simulink model "PlantaHinf"  (R2016a)
settings: Solver=ode45  StartTime=0.0  StopTime=inf  RelTol=1e-3
undefined symbols (not defined in the file or in its folder): K1
libraries: arduino_io_lib x5
settings Model: Creator=Julián  LastModifiedBy=i95sa
settings DataIOCC: LimitDataPoints=on  SaveFormat=Array  SignalLoggingSaveFormat=ModelDataLogs
settings DebuggingCC: SolverPrmCheckMsg=warning  MultiTaskDSMMsg=warning  MultiTaskCondExecSysMsg=none
settings HardwareCC: ProdBitPerPointer=32  ProdLargestAtomicFloat=None  ProdIntDivRoundTo=Undefined  ProdEndianess=Unspecified  ProdWordSize=32  ProdHWDeviceType=32-bit Generic
settings ModelReferenceCC: PropagateSignalLabelsOutOfModel=off
settings ConfigComp: CovModelRefEnable=Off

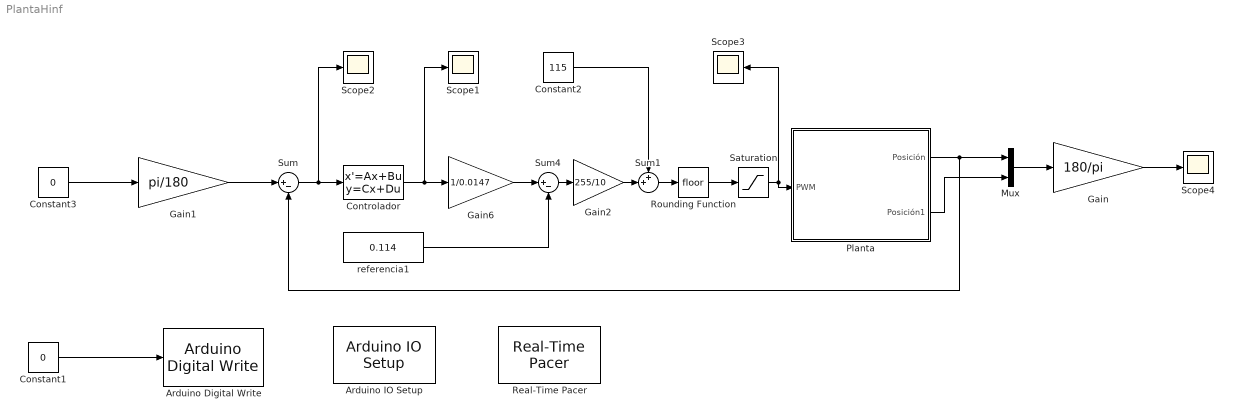
== system PlantaHinf ==
  Arduino Digital Write : arduino_io_lib/Arduino Digital Write  arduinoVar=Existing workspace arduino variable #1  arduinoPin=12  T=0.1
  Arduino IO Setup : arduino_io_lib/Arduino IO Setup  Priority=3  arduinoVar=Existing workspace arduino variable #1  workspaceVarName=ard  comPort=4
  Constant1 : Constant  Value=0
  Constant2 : Constant  Value=115
  Constant3 : Constant  Value=0
  Controlador : StateSpace  A=K1.a  B=K1.b  C=K1.c  D=K1.d  X0=0
  Gain : Gain  Gain=180/pi
  Gain1 : Gain  Gain=pi/180
  Gain2 : Gain  Gain=255/10
  Gain6 : Gain  Gain=1/0.0147
  Mux : Mux  Inputs=2
  Planta : Subsystem
  Real-Time Pacer : arduino_io_lib/Real-Time Pacer  simTimePerRealTime=1
  Rounding Function : Rounding
  Saturation : Saturate  UpperLimit=255  LowerLimit=140
  Scope{1..4} (4 alike) : Scope
  Sum : Sum  Inputs=|+-
  Sum1 : Sum  Inputs=++|
  Sum4 : Sum  Inputs=|+-
  referencia1 : Constant  Value=0.114
  wires:
  Constant3/1 -> Gain1/1
  Sum/1 -> Controlador/1, Scope2/1
  Controlador/1 -> Scope1/1, Gain6/1
  Planta/1(Posición) -> Sum/2, Mux/1
  Gain/1 -> Scope4/1
  Gain1/1 -> Sum/1
  referencia1/1 -> Sum4/2
  Sum4/1 -> Gain2/1
  Sum1/1 -> Rounding Function/1
  Constant1/1 -> Arduino Digital Write/1
  Saturation/1 -> Scope3/1, Planta/1(PWM)
  Constant2/1 -> Sum1/1
  Gain2/1 -> Sum1/2
  Planta/2(Posición1) -> Mux/2
  Mux/1 -> Gain/1
  Gain6/1 -> Sum4/1
  Rounding Function/1 -> Saturation/1

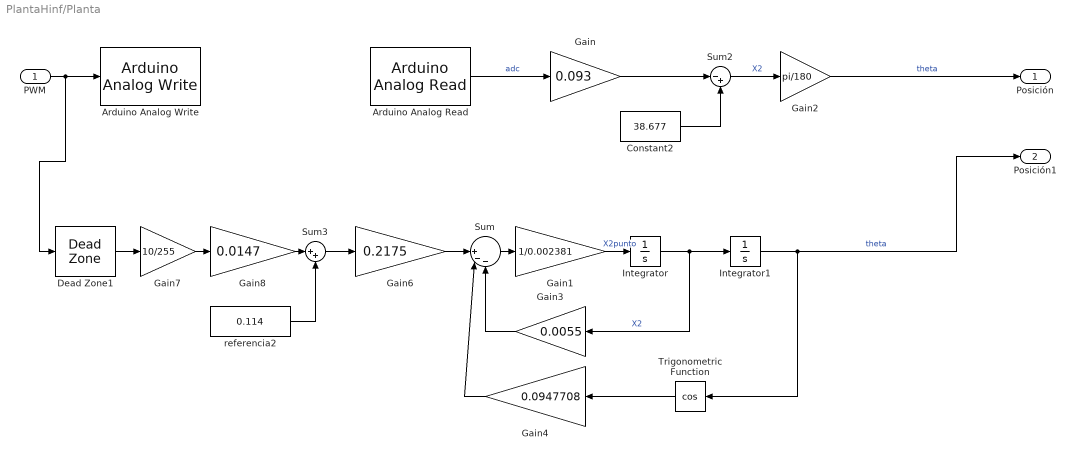
== system PlantaHinf/Planta ==
  PWM : Inport
  Arduino Analog Read : arduino_io_lib/Arduino Analog Read  arduinoVar=Existing workspace arduino variable #1  arduinoPin=8  T=0.1
  Arduino Analog Write : arduino_io_lib/Arduino Analog Write  arduinoVar=Existing workspace arduino variable #1  arduinoPin=3  T=0.1
  Constant2 : Constant  Value=38.677
  Dead Zone1 : DeadZone  LowerValue=0  UpperValue=0  SaturateOnIntegerOverflow=on
  Gain : Gain  Gain=0.093
  Gain1 : Gain  Gain=1/0.002381
  Gain2 : Gain  Gain=pi/180
  Gain3 : Gain  Gain=0.0055
  Gain4 : Gain  Gain=0.0947708
  Gain6 : Gain  Gain=0.2175
  Gain7 : Gain  Gain=10/255
  Gain8 : Gain  Gain=0.0147
  Integrator : Integrator
  Integrator1 : Integrator
  Sum : Sum  Inputs=||+--
  Sum2 : Sum  Inputs=|-+
  Sum3 : Sum  Inputs=|++
  Trigonometric Function : Trigonometry  Operator=cos
  referencia2 : Constant  Value=0.114
  Posición : Outport
  Posición1 : Outport  Port=2
  wires:
  PWM/1 -> Dead Zone1/1, Arduino Analog Write/1
  Arduino Analog Read/1 -> Gain/1  "adc"
  Gain/1 -> Sum2/1
  Constant2/1 -> Sum2/2
  Sum2/1 -> Gain2/1  "X2"
  Gain2/1 -> Posición/1  "theta"
  Sum/1 -> Gain1/1
  Gain1/1 -> Integrator/1  "X2punto"
  Integrator/1 -> Integrator1/1, Gain3/1  "X2"
  Trigonometric Function/1 -> Gain4/1
  Gain3/1 -> Sum/3
  Integrator1/1 -> Posición1/1, Trigonometric Function/1  "theta"
  Gain4/1 -> Sum/2
  Gain6/1 -> Sum/1
  referencia2/1 -> Sum3/2
  Sum3/1 -> Gain6/1
  Gain7/1 -> Gain8/1
  Gain8/1 -> Sum3/1
  Dead Zone1/1 -> Gain7/1
